simulink model "dtc_smo"  (R2023a)
settings: Solver=ode23t  StartTime=0.0  StopTime=T.end  RelTol=1e-3
values from neighbouring files (symbols this model uses):
  A = exp(F*Ts)    [data.m]
  a = exp(-R/L*Ts)    [data.m]
  b = (1-exp(-R*Ts/L))/R    [data.m]
  cutoff_freq = 1200    [data.m]
  eta = 7.8821e-04    (= 0.00078821)    [data.m]
  g = 0.9    [data.m]
  hyst = 0.1    [data.m]
  Ki = 0.1    [data.m]
  Kp = 1.59    [data.m]
  MaxStatorVoltage = 12    [data.m]
  p = 4    [data.m]
  R = Rph_to_ph/2    (= 0.1)    [data.m]
  Ts = 1e-5    (= 1e-05)    [data.m]
  V = 12    [data.m]
  w_max = 10000    [data.m]
undefined symbols (not defined in the file or in its folder): DiscIntNeverNeededParam
libraries: spsMosfetLib x6, mcbcontrolslib x4, mcbsensorlessestimatorlib x4, eeTransforms x3, spsCurrentMeasurementLib x3, spsVoltageMeasurementLib x3, spsGroundLib x2, spsPermanentMagnetSynchronousMachineLib x1, spsDCVoltageSourceLib x1, slpidlib x1, mcbpositiondecoderlib x1, sps_lib x1
settings Model: Creator=Daniil  LastModifiedBy=Daniil
settings DebuggingCC: ParameterPrecisionLossMsg=none
settings RTWCC: GenCodeOnly=on

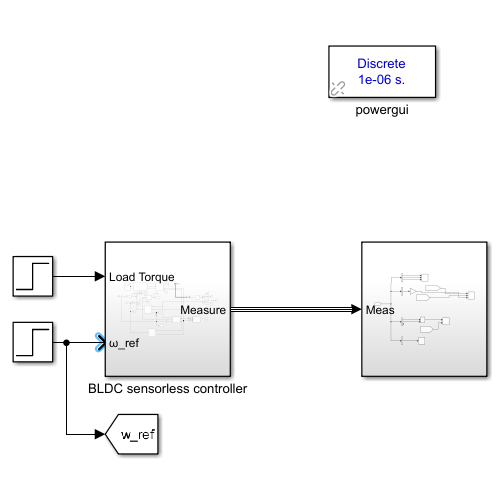
[thumbnail: Simulink's stored preview of the top-level diagram]
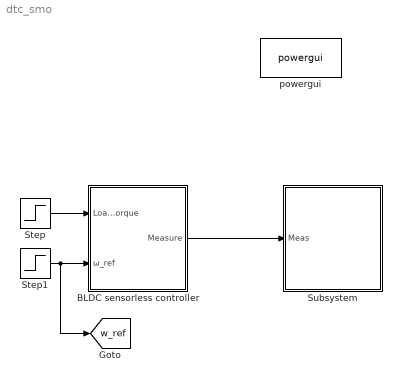
== system dtc_smo ==
  BLDC sensorless controller : Subsystem
  Step : Step  Time=T.end/4  After=0  SampleTime=0
  Step1 : Step  Time=T.end/4  Before=200  After=400  SampleTime=0
  Subsystem : Subsystem
  powergui : sps_lib/powergui  Priority=1  SimulationMode=Discrete  SampleTime=Ts  frequency=60  Iterations=50  frequencyindice=0  Pbase=100e6  ErrMax=1e-4  UnitsV=kV  UnitsW=MW  buscounter=0  FunctionMessages=off  echomessages=off  EnableUseOfTLC=off  CurrentSourceSwitches=off  DisableSnubberDevices=off  DisableRonSwitches=off  DisableVfSwitches=off  DisplayEquations=off  AutomaticDiscreteSolvers=off  SolverType=Tustin/Backward Euler (TBE)  Interpol=off  ExternalGateDelay=off  methode=off  Ts=100  x0status=blocks  SPID=on  SwTol=0  HookPort=off  NonlinearTolerance=1e-4  nMaxIteration=100  ContinueOnMaxIteration=off  RestoreLinks=warning  ResistiveCurrentMeasurement=off  Frange=[0:2:500]  Ylog=off  Xlog=on  ShowGrid=off  save=off  variable=ZData  structure=0  ZoomFFT=off  StartTime=0.0  cycles=1  DisplayStyle=1  fundamental=60  FreqAxis=off  MaxFrequency=1000  frequencyindicesteady=1  RmsSteady=1  display=off
  tag scope: w_ref=global
  wires:
  Step/1 -> BLDC sensorless controller/1(Load Torque)
  Step1/1 -> [w_ref], BLDC sensorless controller/2(ω_ref)
  BLDC sensorless controller/1(Measure) -> Subsystem/1(Meas)

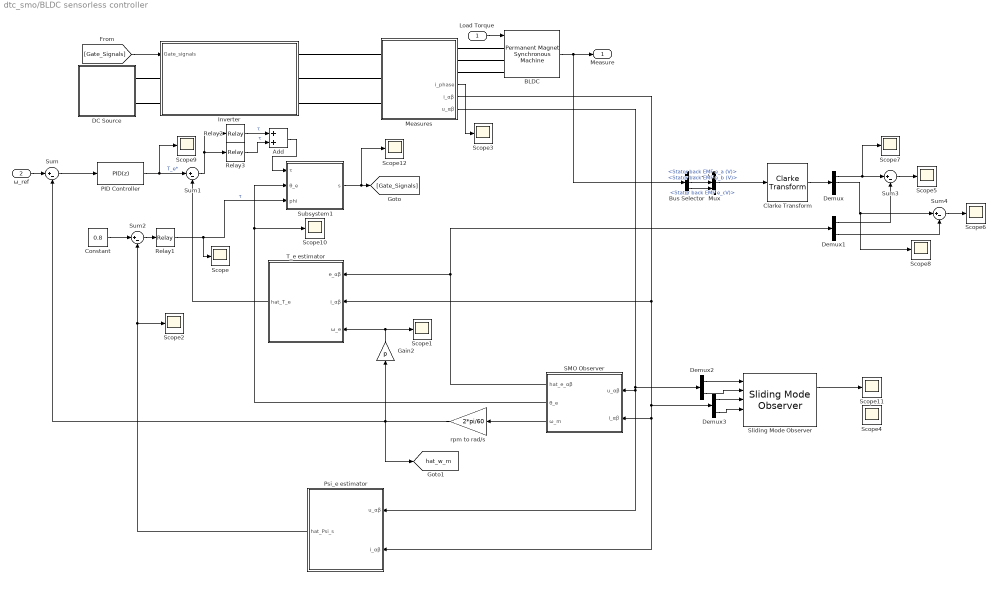
== system dtc_smo/BLDC sensorless controller ==
  Load Torque : Inport
  ω_ref : Inport  Port=2
  Add : Sum
  BLDC : spsPermanentMagnetSynchronousMachineLib/Permanent Magnet Synchronous Machine  NbPhases=3  FluxDistribution=Trapezoidal  RotorType=Round  MechanicalLoad=Torque Tm  PresetModel=No  ShowDetailedParameters=on  MeasurementBus=off  Resistance=0.1  Inductance=0.0225  dqInductances=[8.5e-3,8.5e-3]  La=0.0225  MachineConstant=Flux linkage established by magnets (V.s)  Flux=0.00153463  VoltageCst=1.2856  TorqueCst=0.012277  Flat=120  Mechanical=[3.2141e-07 3.37164e-08 4]  PolePairs=4  InitialConditions=[100,0, 0,0]  InitialConditions5ph=[0 0 0 0 0 0]  RefAngle=90 degrees behind phase A axis (modified Park)  IterativeDiscreteModel=Trapezoidal robust  TsBlock=Ts  TsPowergui=0
  Bus Selector : BusSelector  OutputSignals=Stator back EMF e_a (V),Stator back EMF e_b (V),Stator back EMF e_cV)
  Clarke Transform : eeTransforms/Clarke Transform  PowerInvariant=off
      settings: LibrarySourceBlock=|
      | ee_sl_lib/Mathematical
      | Transforms/Clarke Transform
  Constant : Constant  Value=0.8
  DC Source : Subsystem
  Demux : Demux  Outputs=3
  Demux1 : Demux  Outputs=2
  Demux2 : Demux  Outputs=2
  Demux3 : Demux  Outputs=2
  Gain2 : Gain  Gain=p
  Inverter : Subsystem
  Measures : Subsystem
      settings: PortSchema="{\"entries\":[{\"content\":{\"sides\":[{\"content\":{\"connectorIds\":[\"LConn1\",\"LConn2\",\"LConn3\"]},\"type\":\"ConnectorPlacement.EquallySpacedRectSide\",\"uuid\":\"904635fc-542c-43d3-862b-99e90cc61244\"},{\"content\":{\"connectorIds\":[\"RConn1\",\"RConn2\",\"RConn3\",\"Out1\",\"Out2\",\"Out3\"],\"side\":\"RIGHT\"},\"type\":\"ConnectorPlacement.EquallySpacedRectSide\",\"uuid\":\"d6715f07-2b73-4717-b585-53d74f7e7a63\"},{\"content\":{\"side\":\"TOP\"},\"type\":\"ConnectorPlacement.EquallySpacedRectSide\",\"uuid\":\"35e89841-7e88-4b2f-ad43-54981bf59f97\"}]},\"type\":\"ConnectorPlacement.EquallySpacedConnector\",\"uuid\":\"1a18aced-5813-4034-833a-8e0cb43063d2\"}],\"packageUris\":[\"http://schema.mathworks.com/mf0/Connector/R2020b\"],\"version\":\"1.0\"}"
  Mux : Mux  Inputs=3
  PID Controller : slpidlib/PID Controller  Controller=PID  Form=Parallel  TimeDomain=Discrete-time  UseExternalTs=off  SampleTime=Ts  IntegratorMethod=Forward Euler  FilterMethod=Forward Euler  ControllerParametersSource=internal  P=Kp  I=Ki  UseKiTs=off  D=0  N=100  UseFilter=on  TunerSelectOption=Transfer Function Based (PID Tuner App)  InitialConditionSource=internal  InitialConditionForIntegrator=0  InitialConditionForFilter=0  DifferentiatorICPrevScaledInput=0  ExternalReset=none  TrackingMode=off  Kt=1  LimitOutput=off  SatLimitsSource=internal  UpperSaturationLimit=inf  LowerSaturationLimit=-inf  LinearizeAsGain=on  AntiWindupMode=clamping  Kb=1  LimitIntegrator=off  UpperIntegratorSaturationLimit=10  LowerIntegratorSaturationLimit=-10  POutMin=[]  POutMax=[]  IOutMin=[]  IOutMax=[]  DOutMin=[]  DOutMax=[]  NOutMin=[]  NOutMax=[]  SumOutMin=[]  SumOutMax=[]  SaturationOutMin=[]  SaturationOutMax=[]  PParamMin=[]  PParamMax=[]  IParamMin=[]  IParamMax=[]  DParamMin=[]  DParamMax=[]  NParamMin=[]  NParamMax=[]  KbParamMin=[]  KbParamMax=[]  KtParamMin=[]  KtParamMax=[]  KbOutMin=[]  KbOutMax=[]  KtOutMin=[]  KtOutMax=[]  IntegratorOutMin=[]  IntegratorOutMax=[]  FilterOutMin=[]  FilterOutMax=[]  SumI1OutMin=[]  SumI1OutMax=[]  SumI2OutMin=[]  SumI2OutMax=[]  SumI3OutMin=[]  SumI3OutMax=[]  SumI4OutMin=[]  SumI4OutMax=[]  SumDOutMin=[]  SumDOutMax=[]  DifferentiatorOutMin=[]  DifferentiatorOutMax=[]  FilterDiffOutCoefMin=[]  FilterDiffOutCoefMax=[]  ReciprocalOutMin=[]  ReciprocalOutMax=[]  SumDenOutMin=[]  SumDenOutMax=[]  SumNumOutMin=[]  SumNumOutMax=[]  DivideOutMin=[]  DivideOutMax=[]  UdiffTsProdOutMin=[]  UdiffTsProdOutMax=[]  NTsProdOutMin=[]  NTsProdOutMax=[]  UintegralTsProdOutMin=[]  UintegralTsProdOutMax=[]  UngainTsProdOutMin=[]  UngainTsProdOutMax=[]  ClampingZeroOutDataTypeStr=Inherit: Inherit via back propagation  ClampingZeroOutMin=[]  ClampingZeroOutMax=[]  FilterDenConstantOutDataTypeStr=Inherit: Inherit via back propagation  FilterDenConstantOutMin=[]  FilterDenConstantOutMax=[]  PCopyOutDataTypeStr=Inherit: Inherit via back propagation  PCopyOutMin=[]  PCopyOutMax=[]  NCopyOutDataTypeStr=Inherit: Inherit via back propagation  NCopyOutMin=[]  NCopyOutMax=[]  IntegratorContinuousStateAttributes=''  IntegratorStateMustResolveToSignalObject=off  IntegratorRTWStateStorageClass=Auto  FilterContinuousStateAttributes=''  FilterStateMustResolveToSignalObject=off  FilterRTWStateStorageClass=Auto  ParallelPVariant=InternalParameters  IdealPVariant=Disabled  IVariant=InternalParameters  DVariant=InternalParameters  IntegratorVariant=Discrete  SatVariant=Disabled  AWVariant=Passthrough  PCopyVariant=Disabled  TRVariant=Disabled  FdbkBlocksVariant=Forward  IdealPFdbkVariant=Disabled  SatFdbkVariant=Disabled  DerivativeFilterVariant=ForwardEulerFilter  NVariant=InternalParameters  NCopyVariant=Disabled  FilterICVariant=InternalICsFilter  IntegratorICVariant=InternalICs  ExternalResetVariant=Disabled  TRSumVariant=Passthrough  SumFdbkVariant=Disabled  SumVariant=Sum_PID  TsampFilterVariant=InternalTs  TsampNgainVariant=Passthrough  TsampIntegralVariant=Disabled_SignalSpec  ExternalSaturationOutDataTypeStr=Inherit: Same as second input
  Psi_e estimator : Subsystem
  Relay1 : Relay  OnSwitchValue=hyst/100  OffSwitchValue=-hyst/10  OffOutputValue=-1
  Relay2 : Relay  OnSwitchValue=hyst  OffSwitchValue=0
  Relay3 : Relay  OnSwitchValue=0  OffSwitchValue=-hyst  OnOutputValue=0  OffOutputValue=-1
  SMO Observer : Subsystem
  Scope{,1..12} (13 alike) : Scope
  Sliding Mode Observer : mcbsensorlessestimatorlib/Sliding Mode Observer  InputUnit=SI unit  BlkSampleTime=Ts  StatorResistance=R  StatorInductance=L  MaxApplicationSpeed=10000  PolePairs=4  MaxStatorVoltage=13.8564  MaxStatorCurrent=21.4286  DisturbanceObserverGain=0.9  CurrentObserverGain=3.1529e-06  CutoffFreq=2000  PositionUnit=Degrees  PositionDataType=single  SpeedUnit=Degrees/sec  PerUnitSpeed=6000  SpeedDataType=single
      settings: LibrarySourceBlock=mcblib/Sensorless Estimators/Sliding Mode Observer
  Subsystem1 : Subsystem
  Sum{,1..4} (5 alike) : Sum  Inputs=|+-
  T_e estimator : Subsystem
  rpm to rad/s : Gain  Gain=2*pi/60
  Measure : Outport
  tag scope: hat_w_m=global
  wires:
  Load Torque/1 -> BLDC/1
  BLDC/1 -> Bus Selector/1, Measure/1
  [Gate_Signals] -> Inverter/1(Gate_signals)
  Measures/3(u_αβ) -> Demux2/1, Psi_e estimator/1(u_αβ), SMO Observer/1(u_αβ)
  Measures/2(i_αβ) -> Demux3/1, Psi_e estimator/2(i_αβ), SMO Observer/2(i_αβ), T_e estimator/2(i_αβ)
  Gain2/1 -> T_e estimator/3(ω_e), Scope1/1
  ω_ref/1 -> Sum/1
  Sum/1 -> PID Controller/1
  PID Controller/1 -> Scope9/1, Sum1/1  "T_e*"
  T_e estimator/1(hat_T_e) -> Sum1/2
  Sum1/1 -> Relay3/1, Relay2/1
  Subsystem1/1(s) -> Scope12/1, [Gate_Signals]
  SMO Observer/2(θ_e) -> Scope10/1, Subsystem1/2(θ_e)
  rpm to rad/s/1 -> [hat_w_m], Gain2/1, Sum/2
  SMO Observer/1(hat_e_αβ) -> Demux1/1, T_e estimator/1(e_αβ)
  Measures/1(i_phase) -> Scope3/1
  Sum2/1 -> Relay1/1
  Psi_e estimator/1(hat_Psi_s) -> Scope2/1, Sum2/2
  Constant/1 -> Sum2/1
  Relay1/1 -> Scope/1, Subsystem1/3(phi)  "τ"
  Relay2/1 -> Add/1  "τ"
  Relay3/1 -> Add/2  "τ"
  Add/1 -> Subsystem1/1(τ)
  Bus Selector/1 -> Mux/1  "<Stator back EMF e_a (V)>"
  Bus Selector/2 -> Mux/2  "<Stator back EMF e_b (V)>"
  Bus Selector/3 -> Mux/3  "<Stator back EMF e_cV)>"
  Mux/1 -> Clarke Transform/1
  Clarke Transform/1 -> Demux/1
  Demux/1 -> Scope7/1, Sum3/1
  Demux1/1 -> Sum3/2
  Sum3/1 -> Scope5/1
  Demux/2 -> Scope8/1, Sum4/1
  Demux1/2 -> Sum4/2
  Sum4/1 -> Scope6/1
  Demux2/1 -> Sliding Mode Observer/1
  Demux2/2 -> Sliding Mode Observer/2
  Demux3/1 -> Sliding Mode Observer/3
  Demux3/2 -> Sliding Mode Observer/4
  Sliding Mode Observer/1 -> Scope11/1
  SMO Observer/3(ω_m) -> rpm to rad/s/1
  connections:
  DC Source/RConn1 -- Inverter/LConn1
  DC Source/RConn2 -- Inverter/LConn2
  Measures/LConn1 -- Inverter/RConn1
  Measures/RConn3 -- BLDC/LConn3
  Measures/LConn2 -- Inverter/RConn2
  Measures/LConn3 -- Inverter/RConn3
  Measures/RConn1 -- BLDC/LConn1
  Measures/RConn2 -- BLDC/LConn2

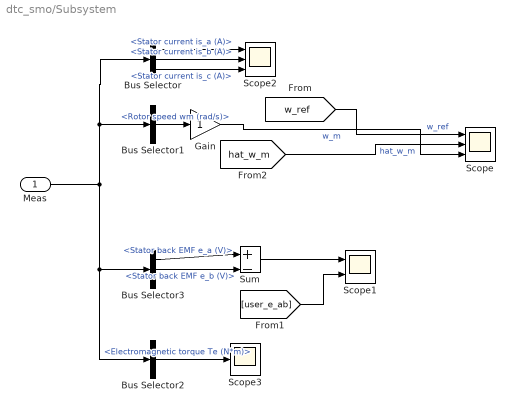
== system dtc_smo/Subsystem ==
  Meas : Inport
  Bus Selector : BusSelector  OutputSignals=Stator current is_a (A),Stator current is_b (A),Stator current is_c (A)
  Bus Selector1 : BusSelector  OutputSignals=Rotor speed wm (rad/s)
  Bus Selector2 : BusSelector  OutputSignals=Electromagnetic torque Te (N*m)
  Bus Selector3 : BusSelector  OutputSignals=Stator back EMF e_a (V),Stator back EMF e_b (V),Stator back EMF e_cV)
  Gain : Gain
  Scope : Scope  NumInputPorts=3
  Scope1 : Scope  NumInputPorts=2
  Scope2 : Scope  NumInputPorts=3
  Scope3 : Scope
  Sum : Sum  Inputs=|+-
  wires:
  Meas/1 -> Bus Selector/1, Bus Selector1/1, Bus Selector3/1, Bus Selector2/1
  Bus Selector3/1 -> Sum/1  "<Stator back EMF e_a (V)>"
  Bus Selector3/2 -> Sum/2  "<Stator back EMF e_b (V)>"
  Sum/1 -> Scope1/1
  [user_e_ab] -> Scope1/2
  Bus Selector/1 -> Scope2/1  "<Stator current is_a (A)>"
  Bus Selector/2 -> Scope2/2  "<Stator current is_b (A)>"
  Bus Selector/3 -> Scope2/3  "<Stator current is_c (A)>"
  Bus Selector2/1 -> Scope3/1  "<Electromagnetic torque Te (N*m)>"
  [w_ref] -> Scope/1  "w_ref"
  Bus Selector1/1 -> Gain/1  "<Rotor speed wm (rad/s)>"
  [hat_w_m] -> Scope/2  "hat_w_m"
  Gain/1 -> Scope/3  "w_m"

== system dtc_smo/BLDC sensorless controller/DC Source ==
  DC Voltage Source : spsDCVoltageSourceLib/DC Voltage Source  Amplitude=V  Measurements=None
  Positive : PMIOPort  Side=Right
  Negaive : PMIOPort  Port=2  Side=Right
  connections:
  DC Voltage Source/LConn1 -- Negaive/RConn1
  DC Voltage Source/RConn1 -- Positive/RConn1

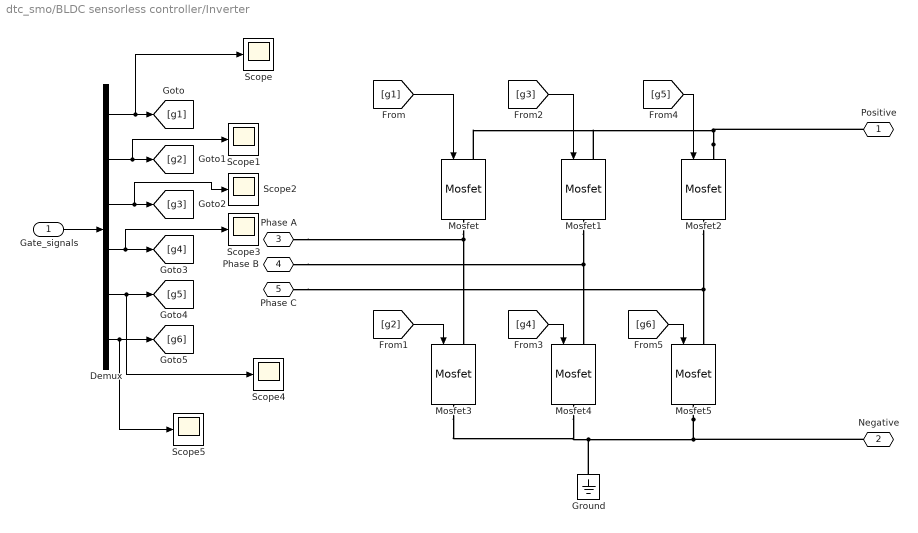
== system dtc_smo/BLDC sensorless controller/Inverter ==
  Gate_signals : Inport
  Demux : Demux  Outputs=6
  Ground : spsGroundLib/Ground  LConnTagsString=a
  Mosfet{,1..5} (6 alike) : spsMosfetLib/Mosfet  Ron=0.0006/95  Lon=0  Rd=0.01  Vfd=0  IC=0  Rs=10e5  Cs=inf  Measurements=off
  Scope{,1..5} (6 alike) : Scope
  Positive : PMIOPort  Side=Left
  Negative : PMIOPort  Port=2  Side=Left
  Phase A : PMIOPort  Port=3  Side=Right
  Phase B : PMIOPort  Port=4  Side=Right
  Phase C : PMIOPort  Port=5  Side=Right
  wires:
  Demux/2 -> Scope1/1, [g2]
  Demux/4 -> Scope3/1, [g4]
  Demux/1 -> Scope/1, [g1]
  [g2] -> Mosfet3/1
  [g3] -> Mosfet1/1
  Demux/5 -> Scope4/1, [g5]
  Demux/6 -> Scope5/1, [g6]
  Gate_signals/1 -> Demux/1
  [g4] -> Mosfet4/1
  [g6] -> Mosfet5/1
  [g5] -> Mosfet2/1
  [g1] -> Mosfet/1
  Demux/3 -> Scope2/1, [g3]
  connections:
  Mosfet5/RConn1 -- Ground/LConn1 -- Mosfet3/RConn1 -- Mosfet4/RConn1 -- Negative/RConn1
  Mosfet2/RConn1 -- Phase C/RConn1 -- Mosfet5/LConn1
  Mosfet1/RConn1 -- Phase B/RConn1 -- Mosfet4/LConn1
  Mosfet/RConn1 -- Phase A/RConn1 -- Mosfet3/LConn1
  Mosfet2/LConn1 -- Positive/RConn1 -- Mosfet/LConn1 -- Mosfet1/LConn1

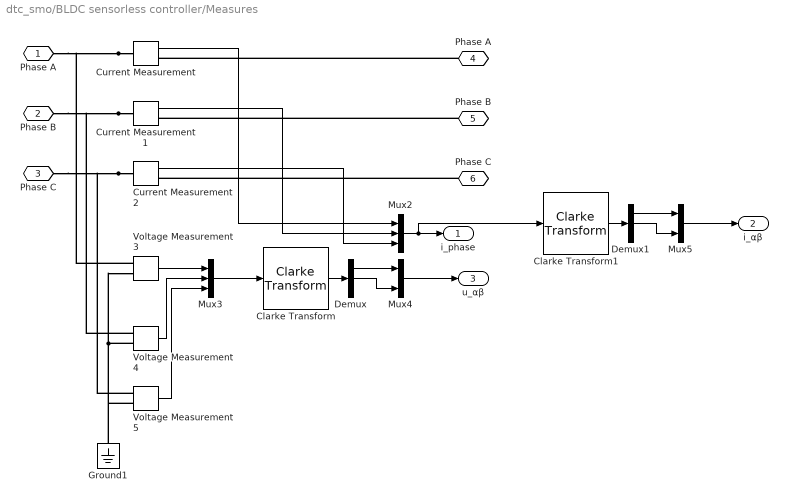
== system dtc_smo/BLDC sensorless controller/Measures ==
  Clarke Transform : eeTransforms/Clarke Transform  PowerInvariant=off
      settings: LibrarySourceBlock=|
      | ee_sl_lib/Mathematical
      | Transforms/Clarke Transform
  Clarke Transform1 : eeTransforms/Clarke Transform  PowerInvariant=off
      settings: LibrarySourceBlock=|
      | ee_sl_lib/Mathematical
      | Transforms/Clarke Transform
  Current Measurement : spsCurrentMeasurementLib/Current Measurement  PhasorSimulation=off  OutputType=Complex  PSBequivalent=0
  Current Measurement1 : spsCurrentMeasurementLib/Current Measurement  PhasorSimulation=off  OutputType=Complex  PSBequivalent=0
  Current Measurement2 : spsCurrentMeasurementLib/Current Measurement  PhasorSimulation=off  OutputType=Complex  PSBequivalent=0
  Demux : Demux  Outputs=3
  Demux1 : Demux  Outputs=3
  Ground1 : spsGroundLib/Ground  LConnTagsString=a
  Mux2 : Mux  Inputs=3
  Mux3 : Mux  Inputs=3
  Mux4 : Mux  Inputs=2
  Mux5 : Mux  Inputs=2
  Voltage Measurement3 : spsVoltageMeasurementLib/Voltage Measurement  PhasorSimulation=off  OutputType=Complex  PSBequivalent=0
  Voltage Measurement4 : spsVoltageMeasurementLib/Voltage Measurement  PhasorSimulation=off  OutputType=Complex  PSBequivalent=0
  Voltage Measurement5 : spsVoltageMeasurementLib/Voltage Measurement  PhasorSimulation=off  OutputType=Complex  PSBequivalent=0
  Phase A : PMIOPort  Side=Left
  Phase B : PMIOPort  Port=2  Side=Left
  Phase C : PMIOPort  Port=3  Side=Left
  "Phase A " : PMIOPort  Port=4  Side=Right
  "Phase B " : PMIOPort  Port=5  Side=Right
  "Phase C " : PMIOPort  Port=6  Side=Right
  i_phase : Outport
  i_αβ : Outport  Port=2
  u_αβ : Outport  Port=3
  wires:
  Current Measurement/1 -> Mux2/1
  Current Measurement2/1 -> Mux2/3
  Mux2/1 -> Clarke Transform1/1, i_phase/1
  Current Measurement1/1 -> Mux2/2
  Voltage Measurement3/1 -> Mux3/1
  Mux3/1 -> Clarke Transform/1
  Voltage Measurement4/1 -> Mux3/2
  Voltage Measurement5/1 -> Mux3/3
  Clarke Transform/1 -> Demux/1
  Demux/1 -> Mux4/1
  Demux/2 -> Mux4/2
  Mux4/1 -> u_αβ/1
  Mux5/1 -> i_αβ/1
  Demux1/1 -> Mux5/1
  Demux1/2 -> Mux5/2
  Clarke Transform1/1 -> Demux1/1
  connections:
  Current Measurement1/LConn1 -- Voltage Measurement4/LConn1 -- Phase B/RConn1
  "Phase B "/RConn1 -- Current Measurement1/RConn1
  Current Measurement/LConn1 -- Phase A/RConn1 -- Voltage Measurement3/LConn1
  "Phase C "/RConn1 -- Current Measurement2/RConn1
  Current Measurement2/LConn1 -- Voltage Measurement5/LConn1 -- Phase C/RConn1
  "Phase A "/RConn1 -- Current Measurement/RConn1
  Voltage Measurement4/LConn2 -- Voltage Measurement3/LConn2 -- Ground1/LConn1 -- Voltage Measurement5/LConn2

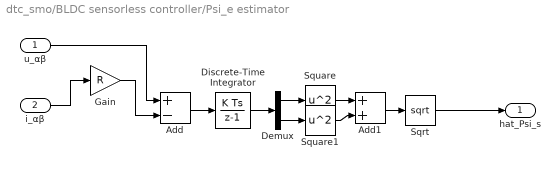
== system dtc_smo/BLDC sensorless controller/Psi_e estimator ==
  u_αβ : Inport
  i_αβ : Inport  Port=2
  Add : Sum  Inputs=+-
  Add1 : Sum
  Demux : Demux  Outputs=2
  Discrete-Time Integrator : DiscreteIntegrator  SampleTime=Ts  ICPrevOutput=DiscIntNeverNeededParam  ICPrevScaledInput=DiscIntNeverNeededParam
  Gain : Gain  Gain=R
  Sqrt : Sqrt
  Square : Math  Operator=square
  Square1 : Math  Operator=square
  hat_Psi_s : Outport
  wires:
  u_αβ/1 -> Add/1
  i_αβ/1 -> Gain/1
  Gain/1 -> Add/2
  Add/1 -> Discrete-Time Integrator/1
  Sqrt/1 -> hat_Psi_s/1
  Discrete-Time Integrator/1 -> Demux/1
  Demux/1 -> Square/1
  Demux/2 -> Square1/1
  Square/1 -> Add1/1
  Square1/1 -> Add1/2
  Add1/1 -> Sqrt/1

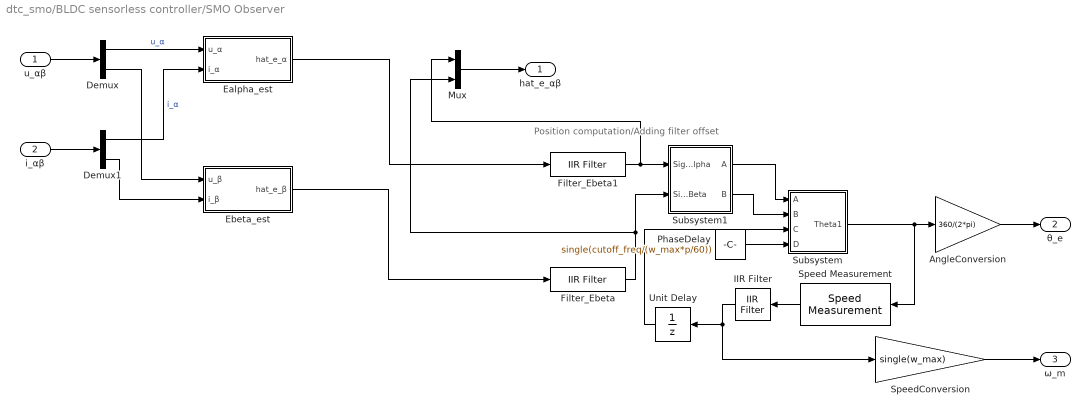
== system dtc_smo/BLDC sensorless controller/SMO Observer ==
  note: Position computation/Adding filter offset
  u_αβ : Inport
  i_αβ : Inport  Port=2
  AngleConversion : Gain  Gain=360/(2*pi)  ParamDataTypeStr=single
  Demux : Demux  Outputs=2
  Demux1 : Demux  Outputs=2
  Ealpha_est : Subsystem
  Ebeta_est : Subsystem
  Filter_Ebeta : mcbcontrolslib/IIR Filter  VariantControl=Low Pass Filter  VariantSelect=Low-pass  Filter_constant=single(2*pi*cutoff_freq*Ts/(2*pi*cutoff_freq*Ts+1))  advancedSettings=on  Ts=Ts  cutOff_freq=1000
  Filter_Ebeta1 : mcbcontrolslib/IIR Filter  VariantControl=Low Pass Filter  VariantSelect=Low-pass  Filter_constant=single(2*pi*cutoff_freq*Ts/(2*pi*cutoff_freq*Ts+1))  advancedSettings=on  Ts=Ts  cutOff_freq=1000
  IIR Filter : mcbcontrolslib/IIR Filter  VariantControl=Low Pass Filter  VariantSelect=Low-pass  Filter_constant=single(Ts*w_max*p/240)  advancedSettings=on  Ts=Ts  cutOff_freq=26.5302
  Mux : Mux  Inputs=2
  PhaseDelay : Constant  Value=single(cutoff_freq/(w_max*p/60))
  Speed Measurement : mcbpositiondecoderlib/Speed Measurement  PositionUnit=Radians  PositionScalingDatatype=uint32  SpeedCalculationMode=Maximum application speed  SampleTimeAsync=Ts  MaximumApplicationSpeed=w_max*p  SpeedResolution=5e-6  DelayLength=749  MaximumMeasurableSpeed=40000  MeasurableSpeedResolution=1.8626e-05  SpeedUnit=Per unit based on dialog  PerUnitSpeed=w_max*p  SpeedDataType=single
  SpeedConversion : Gain  Gain=single(w_max)
  Subsystem : Subsystem
  Subsystem1 : Subsystem
  Unit Delay : UnitDelay  SampleTime=-1  HasFrameUpgradeWarning=on
  hat_e_αβ : Outport
  θ_e : Outport  Port=2  VectorParamsAs1DForOutWhenUnconnected=off
  ω_m : Outport  Port=3  VectorParamsAs1DForOutWhenUnconnected=off
  wires:
  u_αβ/1 -> Demux/1
  i_αβ/1 -> Demux1/1
  Demux/1 -> Ealpha_est/1(u_α)  "u_α"
  Demux1/1 -> Ealpha_est/2(i_α)  "i_α"
  Demux/2 -> Ebeta_est/1(u_β)
  Demux1/2 -> Ebeta_est/2(i_β)
  Subsystem1/1(A) -> Subsystem/1(A)
  Subsystem1/2(B) -> Subsystem/2(B)
  Filter_Ebeta/1 -> Mux/2, Subsystem1/2(SigmaBeta)
  Filter_Ebeta1/1 -> Mux/1, Subsystem1/1(SigmaAlpha)
  Subsystem/1(Theta1) -> Speed Measurement/1, AngleConversion/1
  Speed Measurement/1 -> IIR Filter/1
  PhaseDelay/1 -> Subsystem/4(D)
  Ebeta_est/1(hat_e_β) -> Filter_Ebeta/1
  Unit Delay/1 -> Subsystem/3(C)
  SpeedConversion/1 -> ω_m/1
  IIR Filter/1 -> SpeedConversion/1, Unit Delay/1
  Ealpha_est/1(hat_e_α) -> Filter_Ebeta1/1
  AngleConversion/1 -> θ_e/1
  Mux/1 -> hat_e_αβ/1

== system dtc_smo/BLDC sensorless controller/Subsystem1 ==
  τ : Inport
  θ_e : Inport  Port=2
  phi : Inport  Port=3
  Constant : Constant  Value=360
  MATLAB Function : MATLAB Function  TreatAsAtomicUnit=on
  Mod : Math  Operator=mod
  s : Outport
  wires:
  θ_e/1 -> Mod/1
  Constant/1 -> Mod/2
  MATLAB Function/1(s) -> s/1
  τ/1 -> MATLAB Function/1(tau)
  Mod/1 -> MATLAB Function/3(theta_e)
  phi/1 -> MATLAB Function/2(phi)

== system dtc_smo/BLDC sensorless controller/T_e estimator ==
  e_αβ : Inport
  i_αβ : Inport  Port=2
  ω_e : Inport  Port=3
  Constant : Constant  Value=p
  Demux : Demux  Outputs=2
  Demux1 : Demux  Outputs=2
  MATLAB Function : MATLAB Function  TreatAsAtomicUnit=on
  Scope : Scope
  hat_T_e : Outport
  wires:
  e_αβ/1 -> Demux/1
  i_αβ/1 -> Demux1/1
  Demux/1 -> MATLAB Function/1(e_alpha)
  Demux/2 -> MATLAB Function/2(e_beta)
  Demux1/1 -> MATLAB Function/3(i_alpha)
  Demux1/2 -> MATLAB Function/4(i_beta)
  ω_e/1 -> MATLAB Function/5(w_e)
  Constant/1 -> MATLAB Function/6(p)
  MATLAB Function/1(T_e) -> Scope/1, hat_T_e/1

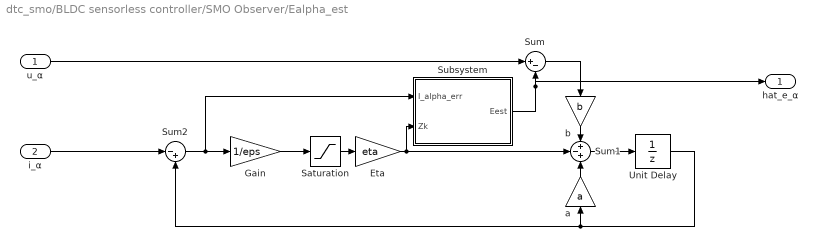
== system dtc_smo/BLDC sensorless controller/SMO Observer/Ealpha_est ==
  u_α : Inport
  i_α : Inport  Port=2
  Eta : Gain  Gain=eta  ParamDataTypeStr=Inherit: Inherit from 'Gain'  OutDataTypeStr=Inherit: Inherit via back propagation  RndMeth=Zero
  Gain : Gain  Gain=1/eps
  Saturation : Saturate  UpperLimit=1  LowerLimit=-1
  Subsystem : Subsystem
  Sum : Sum  Inputs=|+-  OutDataTypeStr=Inherit: Same as first input
  Sum1 : Sum  Inputs=+-+  RndMeth=Zero  OutDataTypeStr=Inherit: Same as first input
  Sum2 : Sum  Inputs=|-+  RndMeth=Zero  OutDataTypeStr=Inherit: Same as first input
  Unit Delay : UnitDelay  SampleTime=Ts  HasFrameUpgradeWarning=on
  a : Gain  Gain=a  ParamDataTypeStr=Inherit: Inherit from 'Gain'  RndMeth=Zero  OutDataTypeStr=Inherit: Same as input
  b : Gain  Gain=b  ParamDataTypeStr=Inherit: Inherit from 'Gain'  RndMeth=Zero  OutDataTypeStr=Inherit: Same as input
  hat_e_α : Outport
  wires:
  Subsystem/1(Eest) -> hat_e_α/1, Sum/2
  Saturation/1 -> Eta/1
  u_α/1 -> Sum/1
  Sum2/1 -> Gain/1, Subsystem/1(I_alpha_err)
  Sum1/1 -> Unit Delay/1
  a/1 -> Sum1/3
  b/1 -> Sum1/1
  i_α/1 -> Sum2/1
  Unit Delay/1 -> Sum2/2, a/1
  Eta/1 -> Sum1/2, Subsystem/2(Zk)
  Sum/1 -> b/1
  Gain/1 -> Saturation/1

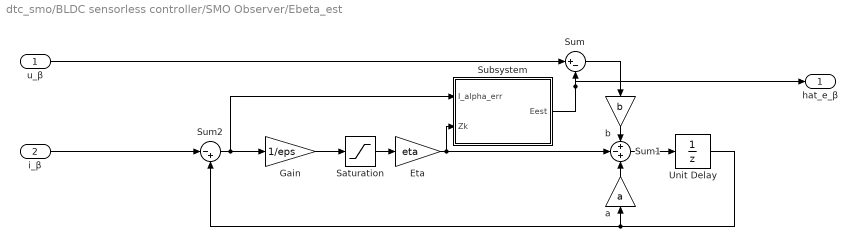
== system dtc_smo/BLDC sensorless controller/SMO Observer/Ebeta_est ==
  u_β : Inport
  i_β : Inport  Port=2
  Eta : Gain  Gain=eta  ParamDataTypeStr=Inherit: Inherit from 'Gain'  OutDataTypeStr=Inherit: Inherit via back propagation  RndMeth=Zero
  Gain : Gain  Gain=1/eps
  Saturation : Saturate  UpperLimit=1  LowerLimit=-1
  Subsystem : Subsystem
  Sum : Sum  Inputs=|+-  OutDataTypeStr=Inherit: Same as first input
  Sum1 : Sum  Inputs=+-+  RndMeth=Zero  OutDataTypeStr=Inherit: Same as first input
  Sum2 : Sum  Inputs=|-+  RndMeth=Zero  OutDataTypeStr=Inherit: Same as first input
  Unit Delay : UnitDelay  SampleTime=Ts  HasFrameUpgradeWarning=on
  a : Gain  Gain=a  ParamDataTypeStr=Inherit: Inherit from 'Gain'  RndMeth=Zero  OutDataTypeStr=Inherit: Same as input
  b : Gain  Gain=b  ParamDataTypeStr=Inherit: Inherit from 'Gain'  RndMeth=Zero  OutDataTypeStr=Inherit: Same as input
  hat_e_β : Outport
  wires:
  Subsystem/1(Eest) -> hat_e_β/1, Sum/2
  u_β/1 -> Sum/1
  Sum1/1 -> Unit Delay/1
  a/1 -> Sum1/3
  b/1 -> Sum1/1
  i_β/1 -> Sum2/1
  Unit Delay/1 -> Sum2/2, a/1
  Eta/1 -> Sum1/2, Subsystem/2(Zk)
  Sum/1 -> b/1
  Gain/1 -> Saturation/1
  Sum2/1 -> Gain/1, Subsystem/1(I_alpha_err)
  Saturation/1 -> Eta/1

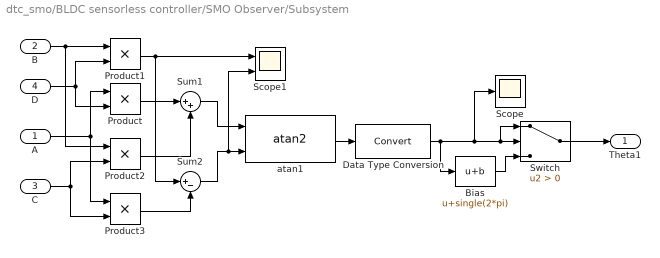
== system dtc_smo/BLDC sensorless controller/SMO Observer/Subsystem ==
  A : Inport
  B : Inport  Port=2
  C : Inport  Port=3
  D : Inport  Port=4
  Bias : Bias  Bias=single(2*pi)  SaturateOnIntegerOverflow=off
  Data Type Conversion : DataTypeConversion  SaturateOnIntegerOverflow=off  RndMeth=Floor
  Product{,1..3} (4 alike) : Product  OutDataTypeStr=Inherit: Inherit via back propagation
  Scope : Scope
  Scope1 : Scope  NumInputPorts=2
  Sum1 : Sum  Inputs=|++  OutDataTypeStr=Inherit: Same as first input
  Sum2 : Sum  Inputs=|+-  OutDataTypeStr=Inherit: Same as first input
  Switch : Switch  Criteria=u2 > Threshold  SaturateOnIntegerOverflow=off  InputSameDT=off
  atan1 : mcbcontrolslib/atan2  outputUnit=Radians
  Theta1 : Outport
  wires:
  D/1 -> Product1/2, Product/2
  B/1 -> Product1/1, Product2/1
  atan1/1 -> Data Type Conversion/1
  Sum1/1 -> atan1/1
  Product/1 -> Sum1/1
  C/1 -> Product3/2, Product2/2
  A/1 -> Product3/1, Product/1
  Switch/1 -> Theta1/1
  Bias/1 -> Switch/3
  Sum2/1 -> Scope1/2, atan1/2
  Data Type Conversion/1 -> Bias/1, Scope/1, Switch/2, Switch/1
  Product1/1 -> Scope1/1, Sum2/1
  Product2/1 -> Sum1/2
  Product3/1 -> Sum2/2

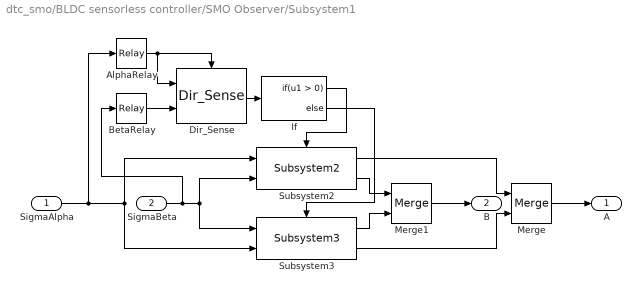
== system dtc_smo/BLDC sensorless controller/SMO Observer/Subsystem1 ==
  SigmaAlpha : Inport
  SigmaBeta : Inport  Port=2
  AlphaRelay : Relay  OnSwitchValue=MaxStatorVoltage*0.02  OffSwitchValue=-MaxStatorVoltage*0.02  OutDataTypeStr=boolean
  BetaRelay : Relay  OnSwitchValue=MaxStatorVoltage*0.02  OffSwitchValue=-MaxStatorVoltage*0.02  OutDataTypeStr=boolean
  Dir_Sense : mcbsensorlessestimatorlib/Sliding Mode Observer/Direction_Latch/Dir_Sense  SystemSampleTime=-1  VariantActivationTime=update diagram  Latency=0  AutoFrameSizeCalculation=off
  If : If
  Merge : Merge
  Merge1 : Merge
  Subsystem2 : mcbsensorlessestimatorlib/Sliding Mode Observer/Direction_Latch/Subsystem2  SystemSampleTime=-1  VariantActivationTime=update diagram  Latency=0  AutoFrameSizeCalculation=off
  Subsystem3 : mcbsensorlessestimatorlib/Sliding Mode Observer/Direction_Latch/Subsystem3  SystemSampleTime=-1  VariantActivationTime=update diagram  Latency=0  AutoFrameSizeCalculation=off
  A : Outport
  B : Outport  Port=2
  wires:
  SigmaAlpha/1 -> Subsystem3/2, Subsystem2/1, AlphaRelay/1
  Subsystem2/1 -> Merge/1
  If/1 -> Subsystem2/Action
  If/2 -> Subsystem3/Action
  AlphaRelay/1 -> Dir_Sense/1, Dir_Sense/Trigger
  BetaRelay/1 -> Dir_Sense/2
  Merge1/1 -> B/1
  Subsystem3/2 -> Merge/2
  Merge/1 -> A/1
  Subsystem2/2 -> Merge1/1
  Dir_Sense/1 -> If/1
  Subsystem3/1 -> Merge1/2
  SigmaBeta/1 -> Subsystem2/2, Subsystem3/1, BetaRelay/1

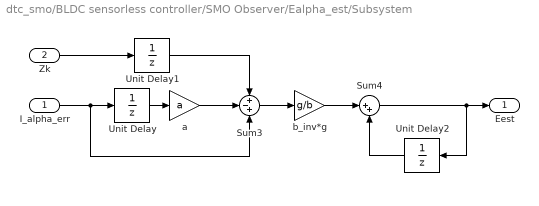
== system dtc_smo/BLDC sensorless controller/SMO Observer/Ealpha_est/Subsystem ==
  I_alpha_err : Inport
  Zk : Inport  Port=2
  Sum3 : Sum  Inputs=+-+  OutDataTypeStr=Inherit: Inherit via back propagation  RndMeth=Zero
  Sum4 : Sum  Inputs=|++  OutDataTypeStr=Inherit: Inherit via back propagation  RndMeth=Zero
  Unit Delay : UnitDelay  SampleTime=Ts  HasFrameUpgradeWarning=on
  Unit Delay1 : UnitDelay  SampleTime=Ts  HasFrameUpgradeWarning=on
  Unit Delay2 : UnitDelay  SampleTime=Ts  HasFrameUpgradeWarning=on
  a : Gain  Gain=a  ParamDataTypeStr=Inherit: Inherit from 'Gain'  RndMeth=Zero  OutDataTypeStr=Inherit: Same as input
  b_inv*g : Gain  Gain=g/b  ParamDataTypeStr=Inherit: Inherit from 'Gain'  RndMeth=Zero  OutDataTypeStr=Inherit: Same as input
  Eest : Outport
  wires:
  Sum3/1 -> b_inv*g/1
  Sum4/1 -> Unit Delay2/1, Eest/1
  Unit Delay/1 -> a/1
  I_alpha_err/1 -> Unit Delay/1, Sum3/3
  Zk/1 -> Unit Delay1/1
  a/1 -> Sum3/2
  Unit Delay2/1 -> Sum4/2
  Unit Delay1/1 -> Sum3/1
  b_inv*g/1 -> Sum4/1

== system dtc_smo/BLDC sensorless controller/SMO Observer/Ebeta_est/Subsystem ==
  I_alpha_err : Inport
  Zk : Inport  Port=2
  Sum3 : Sum  Inputs=+-+  OutDataTypeStr=Inherit: Inherit via back propagation  RndMeth=Zero
  Sum4 : Sum  Inputs=|++  OutDataTypeStr=Inherit: Inherit via back propagation  RndMeth=Zero
  Unit Delay : UnitDelay  SampleTime=Ts  HasFrameUpgradeWarning=on
  Unit Delay1 : UnitDelay  SampleTime=Ts  HasFrameUpgradeWarning=on
  Unit Delay2 : UnitDelay  SampleTime=Ts  HasFrameUpgradeWarning=on
  a1 : Gain  Gain=a  ParamDataTypeStr=Inherit: Inherit from 'Gain'  RndMeth=Zero  OutDataTypeStr=Inherit: Same as input
  b_inv*g : Gain  Gain=g/b  ParamDataTypeStr=Inherit: Inherit from 'Gain'  RndMeth=Zero  OutDataTypeStr=Inherit: Same as input
  Eest : Outport
  wires:
  Sum3/1 -> b_inv*g/1
  Sum4/1 -> Unit Delay2/1, Eest/1
  Unit Delay/1 -> a1/1
  I_alpha_err/1 -> Unit Delay/1, Sum3/3
  Zk/1 -> Unit Delay1/1
  a1/1 -> Sum3/2
  Unit Delay2/1 -> Sum4/2
  Unit Delay1/1 -> Sum3/1
  b_inv*g/1 -> Sum4/1

== matlab function dtc_smo/BLDC sensorless controller/Subsystem1/MATLAB Function ==
  data: tau input; phi input; s output; theta_e input
function s = fcn(tau, phi, theta_e)

V1 = [1, 0, 0, 0, 0, 1]';
V2 = [0, 0, 1, 0, 0, 1]';
V3 = [0, 1, 1, 0, 0, 0]';
V4 = [0, 1, 0, 0, 1, 0]';
V5 = [0, 0, 0, 1, 1, 0]';
V6 = [1, 0, 0, 1, 0, 0]';

if phi == 1
    if tau == 1
        if theta_e >= 0 && theta_e <= 30 || theta_e > 330
            s = V2;
        else if theta_e > 30 && theta_e <= 90
            s = V3;
        else if theta_e > 90 && theta_e <= 150
            s = V4;
        else if theta_e > 150 && theta_e <= 210
            s = V5;
        else if theta_e > 210 && theta_e <= 270
            s = V6;
        else if theta_e > 270 && theta_e <= 330
            s = V1;
        else
            s = zeros(6,1);
        end
        end
        end
        end
        end
        end
    else
        if theta_e >= 0 && theta_e <= 30 || theta_e > 330
            s = V6;
        else if theta_e > 30 && theta_e <= 90
            s = V1;
        else if theta_e > 90 && theta_e <= 150
            s = V2;
        else if theta_e > 150 && theta_e <= 210
            s = V3;
        else if theta_e > 210 && theta_e <= 270
            s = V4;
        else if theta_e > 270 && theta_e <= 330
            s = V5;
        else
            s = zeros(6,1);
        end
        end
        end
        end
        end
        end
    end
else
    if tau == 1
        if theta_e >= 0 && theta_e <= 30 || theta_e > 330
            s = V3;
        else if theta_e > 30 && theta_e <= 90
            s = V4;
        else if theta_e > 90 && theta_e <= 150
            s = V5;
        else if theta_e > 150 && theta_e <= 210
            s = V6;
        else if theta_e > 210 && theta_e <= 270
            s = V1;
        else if theta_e > 270 && theta_e <= 330
            s = V2;
        else
            s = zeros(6,1);
        end
        end
        end
        end
        end
        end
    else
        if theta_e >= 0 && theta_e <= 30 || theta_e > 330
            s = V5;
        else if theta_e > 30 && theta_e <= 90
            s = V6;
        else if theta_e > 90 && theta_e <= 150
            s = V1;
        else if theta_e > 150 && theta_e <= 210
            s = V2;
        else if theta_e > 210 && theta_e <= 270
            s = V3;
        else if theta_e > 270 && theta_e <= 330
            s = V4;
        else
            s = zeros(6,1);
        end
        end
        end
        end
        end
        end
    end

end

== matlab function dtc_smo/BLDC sensorless controller/T_e estimator/MATLAB Function ==
  data: e_alpha input; T_e output; e_beta input; i_alpha input; i_beta input; w_e input; p input
function T_e = fcn(e_alpha, e_beta, i_alpha, i_beta, w_e, p)

T_e = 3*p/4*(e_alpha*i_alpha/w_e+e_beta/w_e*i_beta);
